simulink model "LinearMfObsv"  (R2017a)
settings: Solver=FixedStepAuto  StartTime=0.0  StopTime=10  FixedStep=0.01  RelTol=1e-3
values from neighbouring files (symbols this model uses):
  A = double([ 0, 0, 1, 0; 0, 0, 0, 1; A11, A12, A13, A14;     A21, A22, A23, A24])    [FurutaConstants.m]    (also in axbu.m = [ 0, 0, 1, 0; 0, 0, 0, 1; A11, A12, A13, A14; A21, A22, A23,)
  B = double([0; 0; B1; B2])    [FurutaConstants.m]    (also in axbu.m = [0; 0; B1; B2])
  C1 = Eq1 - H11*ddtheta1 - H12*ddtheta2 - G1    [Code.m]    (also in FurutaConstants.m = [ 1 0 0 0 ]; FurutaSymbolic.m)
  C2 = simplify(Eq2 - H21*ddtheta1 - H22*ddtheta2 - G2)    [Code.m]    (also in FurutaConstants.m = [ 0 1 0 0 ]; FurutaSymbolic.m)
  dtheta1o = 0    [FurutaConstants.m]
  dtheta2o = 0    [FurutaConstants.m]
  K = [0 0 0 1]*(inv(M))*Phi    [Ackermanns.m]    (also in FurutaConstants.m = place(A,B,poles1))
  theta1o = 0    [FurutaConstants.m]
  theta2o = 14*pi/180    (= 0.244346095279)    [FurutaConstants.m]
settings Model: Creator=felip  LastModifiedBy=felip

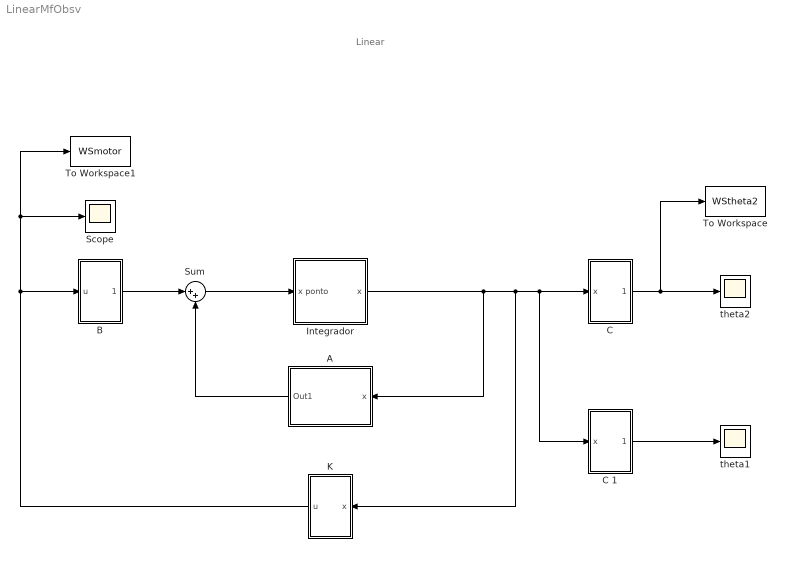
== system LinearMfObsv ==
  note: Linear
  "A " : Subsystem
  "B " : Subsystem
  "C " : Subsystem
  C 1 : Subsystem
  Integrador : Subsystem
  "K " : Subsystem
  Scope : Scope
  Sum : Sum  Inputs=|++
  To Workspace : ToWorkspace  VariableName=WStheta2  SaveFormat=Timeseries  SampleTime=-1
  To Workspace1 : ToWorkspace  VariableName=WSmotor  SaveFormat=Timeseries  SampleTime=-1
  theta1 : Scope
  "theta2 " : Scope
  wires:
  "B "/1(Out1) -> Sum/1
  "A "/1(Out1) -> Sum/2
  Integrador/1(x) -> "K "/1(x), C 1/1(x), "C "/1(x), "A "/1(x)
  C 1/1(theta2) -> theta1/1
  "K "/1(u) -> Scope/1, To Workspace1/1, "B "/1(u)
  "C "/1(theta2) -> To Workspace/1, "theta2 "/1
  Sum/1 -> Integrador/1(x ponto)

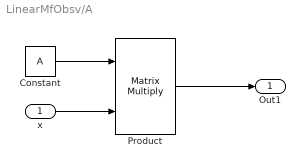
== system LinearMfObsv/A  ==
  x : Inport
  Constant : Constant  Value=A  VectorParams1D=off
  Product : Product  Multiplication=Matrix(*)
  Out1 : Outport
  wires:
  x/1 -> Product/2
  Product/1 -> Out1/1
  Constant/1 -> Product/1

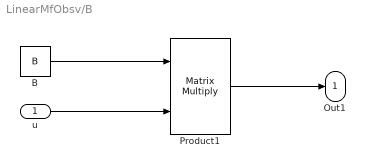
== system LinearMfObsv/B  ==
  u : Inport
  B : Constant  Value=B  VectorParams1D=off
  Product1 : Product  Multiplication=Matrix(*)
  Out1 : Outport
  wires:
  Product1/1 -> Out1/1
  u/1 -> Product1/2
  B/1 -> Product1/1

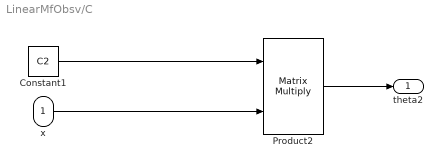
== system LinearMfObsv/C  ==
  x : Inport
  Constant1 : Constant  Value=C2  VectorParams1D=off
  Product2 : Product  Multiplication=Matrix(*)
  theta2 : Outport
  wires:
  x/1 -> Product2/2
  Product2/1 -> theta2/1
  Constant1/1 -> Product2/1

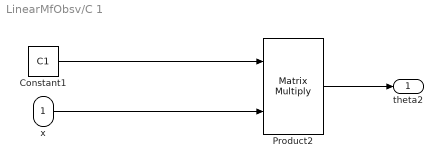
== system LinearMfObsv/C 1 ==
  x : Inport
  Constant1 : Constant  Value=C1  VectorParams1D=off
  Product2 : Product  Multiplication=Matrix(*)
  theta2 : Outport
  wires:
  x/1 -> Product2/2
  Product2/1 -> theta2/1
  Constant1/1 -> Product2/1

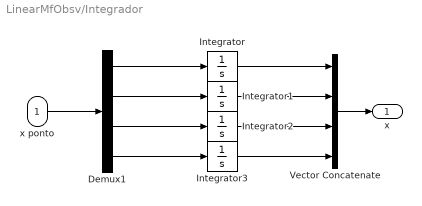
== system LinearMfObsv/Integrador ==
  x ponto : Inport
  Demux1 : Demux
  Integrator : Integrator  InitialCondition=theta1o
  Integrator1 : Integrator  InitialCondition=theta2o
  Integrator2 : Integrator  InitialCondition=dtheta1o
  Integrator3 : Integrator  InitialCondition=dtheta2o
  Vector Concatenate : Concatenate  NumInputs=4  ConcatenateDimension=4
  x : Outport
  wires:
  Demux1/2 -> Integrator1/1
  Demux1/4 -> Integrator3/1
  Demux1/3 -> Integrator2/1
  Integrator/1 -> Vector Concatenate/1
  Integrator2/1 -> Vector Concatenate/3
  Demux1/1 -> Integrator/1
  Integrator3/1 -> Vector Concatenate/4
  Integrator1/1 -> Vector Concatenate/2
  x ponto/1 -> Demux1/1
  Vector Concatenate/1 -> x/1

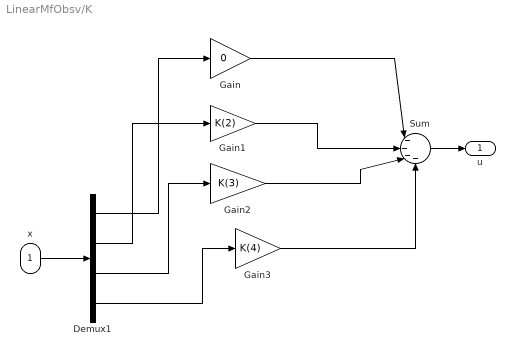
== system LinearMfObsv/K  ==
  x : Inport
  Demux1 : Demux
  Gain : Gain  Gain=0
  Gain1 : Gain  Gain=K(2)
  Gain2 : Gain  Gain=K(3)
  Gain3 : Gain  Gain=K(4)
  Sum : Sum  Inputs=|----
  u : Outport
  wires:
  Sum/1 -> u/1
  x/1 -> Demux1/1
  Demux1/1 -> Gain/1
  Demux1/2 -> Gain1/1
  Demux1/3 -> Gain2/1
  Demux1/4 -> Gain3/1
  Gain/1 -> Sum/1
  Gain1/1 -> Sum/2
  Gain2/1 -> Sum/3
  Gain3/1 -> Sum/4
